simulink model "sim12ex11"  (Simulink 2.09)
settings: Solver=ode45  StartTime=0.0  StopTime=2  MaxStep=.010  RelTol=1e-3  AbsTol=1e-3
values from neighbouring files (symbols this model uses):
  k = 10    [EXA21.M]    (also in FRQLAG.M = 1; FRQLEAD.M = 1)
settings Model: SaveTime=off  SaveOutput=off  ConsistencyChecking=off  RTWTemplateMakefile=grt_vc.tmf

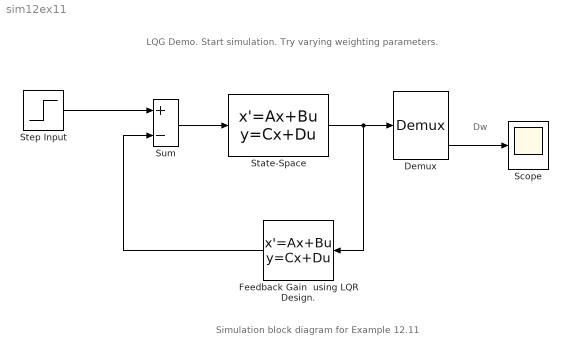
== system sim12ex11 ==
  note: Simulation block diagram for Example 12.11
  note: Dw
  note: LQG Demo. Start simulation.
      | Try varying weighting parameters.
  Demux : Demux  Outputs=3
  Feedback Gain  using LQR Design. : StateSpace  Orientation=left  A=[]  B=[]  C=[]  D=k  X0=0  mask(Regulator){@1=[-5   0   -100;  2   -2    0;   0    0.1   -0.08], @2=[0;   0;    -0.1], @3=eye(3), @4=zeros(3,1), @5=[20, 0  0;  0  10   0;  0   0   5], @6=eye(1,1)*.15}
      mask prompts: @1 "Plant A matrix:"; @2 "Plant B matrix:"; @3 "Plant C matrix:"; @4 "Plant D matrix:"; @5 "Output weighting, y'Qy:"; @6 "Input weighting, u'Ru:"
      mask help:
      | Linear quadratic regulator.
      | (Requires Control Toolbox)
      mask init:
      | [k]=lqry(@1,@2,@3,@4,@5,@6);
      mask Help: Implements a linear state quadratic regulator. Mask and unmask this block to see how it works.
      mask Display: disp('K')
  Scope : Scope
      settings: TickLabels=on  TimeRange=auto  YMin=-5  YMax=5  SaveToWorkspace=off  SaveName=ScopeData
  State-Space : StateSpace  A="[-5  0  -100;  2  -2  0;  0  0.1  -0.08]"  B="[0;   0 ;  -0.1]"  C=eye(3)  D=zeros(3, 1)  X0=0
  Step Input : Step  Time=10  Before=0.2  After=.2
  Sum : Sum  Inputs=+-
  wires:
  Sum/1 -> State-Space/1
  Step Input/1 -> Sum/1
  Demux/3 -> Scope/1
  State-Space/1 -> Demux/1, Feedback Gain  using LQR Design./1
  Feedback Gain  using LQR Design./1 -> Sum/2
